simulink library "Lib_Cntrl_SimplePIcontroller_TMATS_org"  (Simulink 10.0)
settings: Solver=ode45  StartTime=0.0  StopTime=10.0  RelTol=1e-3  EnableMultiTasking=on
Description:
  | Thomas Modules
settings Model: Creator=jwchapm2  LastModifiedBy=annonymous

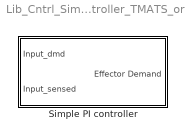
== system Lib_Cntrl_SimplePIcontroller_TMATS_org ==
  Simple PI controller : Subsystem  mask(T-MATS: Simple PI controller Library Block){Kp_M=0.05, Ki_M=0.1, PI_IC_M=70}
      mask prompts: Kp_M "Kp_M - Proportional Gain"; Ki_M "Ki_M - Intragrator Gain"; PI_IC_M "PI_IC_M - PI initial condition"
      mask help:
      | Simple PI contoroller:
      | DMD - Sens = Error
      | Error*(Kp + Ki/s) = Effector DMD
      mask Help: web(which('Control_TMATS_PIC.html'),'-helpbrowser')

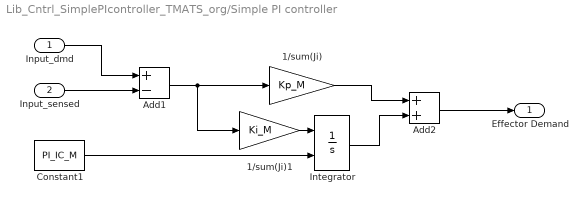
== system Lib_Cntrl_SimplePIcontroller_TMATS_org/Simple PI controller ==
  Input_dmd : Inport
  Input_sensed : Inport  Port=2
  1/sum(Ji) : Gain  Gain=Kp_M  SaturateOnIntegerOverflow=on  OutDataTypeStr=Inherit: Same as input  ParamDataTypeStr=Inherit: Same as input
  1/sum(Ji)1 : Gain  Gain=Ki_M  SaturateOnIntegerOverflow=on  OutDataTypeStr=Inherit: Same as input  ParamDataTypeStr=Inherit: Same as input
  Add1 : Sum  Inputs=+-
  Add2 : Sum
  Constant1 : Constant  Value=PI_IC_M
  Integrator : Integrator  InitialConditionSource=external
  Effector Demand : Outport
  wires:
  Add1/1 -> 1/sum(Ji)/1, 1/sum(Ji)1/1
  Input_sensed/1 -> Add1/2
  1/sum(Ji)/1 -> Add2/1
  Input_dmd/1 -> Add1/1
  Integrator/1 -> Add2/2
  Constant1/1 -> Integrator/2
  1/sum(Ji)1/1 -> Integrator/1
  Add2/1 -> Effector Demand/1
